simulink model "GridTiedInverterOptimalI_2024_SS"  (R2024a)
settings: Solver=ode23t  StartTime=0  StopTime=0.35  FixedStep=Ts  RelTol=1e-3  EnableMultiTasking=on
PreLoadFcn:
  | GridTiedInverterOptimalIData;
undefined symbols (not defined in the file or in its folder): Ad, Bd, K, Ts, Tsc
libraries: eeTransforms x3, eeLuenbergerObserver x1, eePwmGeneratorTwoLevel x1, eeSinusoidalMeasurement x1, SignalEditorBlockLib x1
CloseFcn:
  | try,close(h1_GridTiedInverterOptimalI),end
  | clear h1_GridTiedInverterOptimalI
  | 
  | 
  | clear simlog_GridTiedInverterOptimalI
  | clear logsout_GridTiedInverterOptimalI
  | 
  | clear Ad Ae Bd Be Cd Ce Dd De Lf Rf
  | clear K L omega Ts  Tsc fsw
Description:
  | Three-Phase Grid-Tied Inverter Optimal Current Control
settings Model: Creator=The MathWorks, Inc.  LastModifiedBy=dilu2
settings SolverCC: AlgebraicLoopSolver=TrustRegion  MaxZcPerStep=1
settings DataIOCC: SaveFormat=Array  SaveOutput=off  SaveTime=off  ReturnWorkspaceOutputs=off  SignalLoggingName=logsout_GridTiedInverterOptimalI
settings OptimizationCC: ReuseModelBlockBuffer=off  ExpressionDepthLimit=2147483647  LifeSpan=inf
settings DebuggingCC: UnconnectedInputMsg=warning  UnconnectedOutputMsg=warning  UnconnectedLineMsg=warning  AllowSymbolicDim=off  StateNameClashWarn=warning  SFUnexpectedBacktrackingDiag=warning  SFNoUnconditionalDefaultTransitionDiag=warning  SFExecutionAtInitializationDiag=none  ArithmeticOperatorsInVariantConditions=warning
settings HardwareCC: ProdBitPerPointer=32  ProdBitPerSizeT=32  ProdBitPerPtrDiffT=32  ProdLargestAtomicFloat=None  ProdIntDivRoundTo=Undefined  ProdEndianess=Unspecified  ProdWordSize=32  ProdHWDeviceType=32-bit Generic
settings ModelReferenceCC: EnableRefExpFcnMdlSchedulingChecks=on  PropagateSignalLabelsOutOfModel=off
settings SFSimCC: SimUseLocalCustomCode=off  CustomCodeUndefinedFunction=UseInterfaceOnly
settings RTWCC: RTWUseLocalCustomCode=off  GPUComputeCapability=3.5  DLArmComputeVersion=19.05
settings CodeAppCC: StateflowObjectComments=on
settings GRTTargetCC: TargetLangStandard=C89/C90 (ANSI)  CombineOutputUpdateFcns=off  GRTInterface=on
settings ConfigComp: CovMetricSettings=dw  CovSaveCumulativeToWorkspaceVar=on  CovSaveSingleToWorkspaceVar=on  CovExternalEMLEnable=off
settings SimscapeCC: SimscapeNormalizeSystem=off  SimscapeLogName=simlog_GridTiedInverterOptimalI

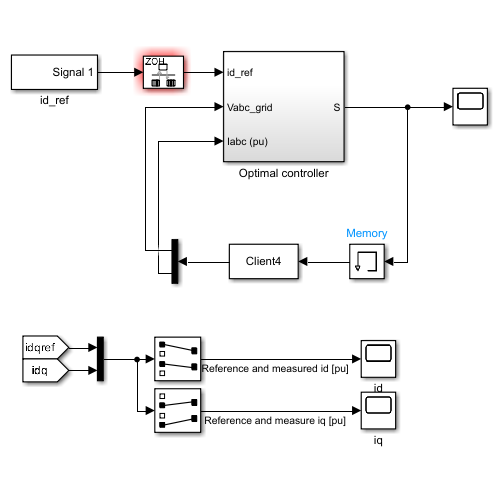
[thumbnail: Simulink's stored preview of the top-level diagram]
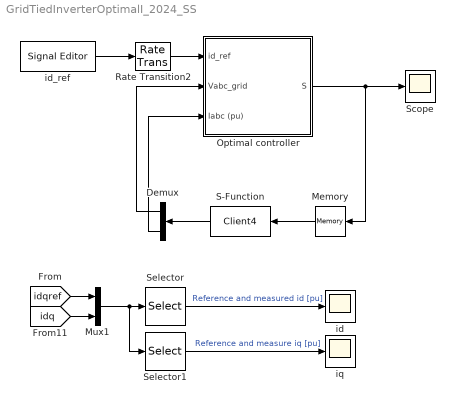
== system GridTiedInverterOptimalI_2024_SS ==
  Demux : Demux  Outputs=2
  Memory : Memory
  Mux1 : Mux  Inputs=2
  Optimal controller : Subsystem
  Rate Transition2 : RateTransition  OutPortSampleTime=Tsc
  S-Function : S-Function  FunctionName=Client4  SFunctionDeploymentMode=off  EnableBusSupport=off
  Scope : Scope
  Selector : Selector  InputPortWidth=4  IndexOptions=Index vector (dialog)  Indices=[1 3]  OutputSizes=1
  Selector1 : Selector  InputPortWidth=4  IndexOptions=Index vector (dialog)  Indices=[2 4]  OutputSizes=1
  id : Scope
  id_ref : SignalEditorBlockLib/Signal Editor  FileName=GridTiedInverterOptimalIIdReference.mat  ActiveScenario=Group_1  ActiveSignal=Signal 1  IsBus=off  OutputBusObjectStr=Bus: BusObject  SampleTime=0  OutputAfterFinalValue=Extrapolation  Unit=inherit  PreserveSignalName=on  ApplySigPropsToAllScenarios=on  ApplySigPropsToAllSignals=off
  iq : Scope
  wires:
  id_ref/1 -> Rate Transition2/1
  Rate Transition2/1 -> Optimal controller/1(id_ref)
  Demux/1 -> Optimal controller/2(Vabc_grid)
  Demux/2 -> Optimal controller/3(Iabc (pu))
  S-Function/1 -> Demux/1
  Optimal controller/1(S) -> Memory/1, Scope/1
  Mux1/1 -> Selector1/1, Selector/1
  Selector/1 -> id/1  "Reference and measured id [pu]"
  [idq] -> Mux1/2
  [idqref] -> Mux1/1
  Selector1/1 -> iq/1  "Reference and measure iq [pu]"
  Memory/1 -> S-Function/1

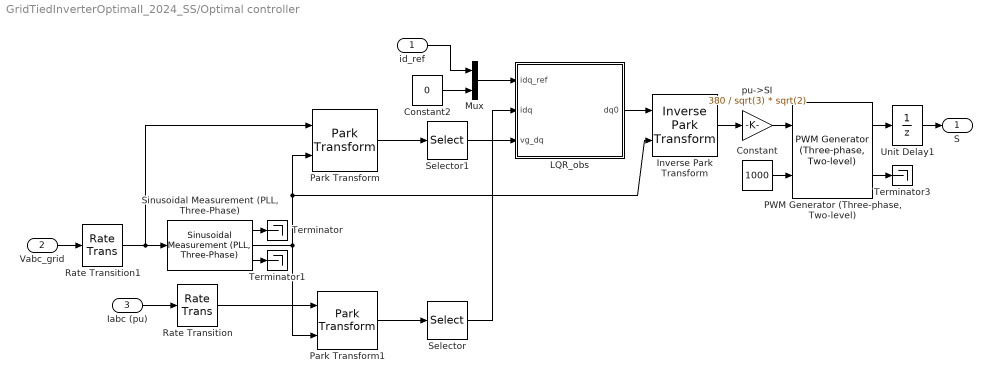
== system GridTiedInverterOptimalI_2024_SS/Optimal controller ==
  id_ref : Inport
  Vabc_grid : Inport  Port=2
  Iabc (pu) : Inport  Port=3
  Constant : Constant  Value=1000
  Constant2 : Constant  Value=0  SampleTime=Tsc
  Inverse Park Transform : eeTransforms/Inverse Park Transform  AxisAlignment=Q-axis  PowerInvariant=off
  LQR_obs : Subsystem
  Mux : Mux  Inputs=2
  "PWM Generator (Three-phase, Two-level)" : eePwmGeneratorTwoLevel/PWM Generator (Three-phase, Two-level)  PWMMode=Continuous PWM (CPWM)  CPWMMode=SPWM: sinusoidal PWM  DPWMMode=60 DPWM: 60 degree discontinuous PWM  fsw=10000  Ts=Ts
  Park Transform : eeTransforms/Park Transform  AxisAlignment=Q-axis  PowerInvariant=off
  Park Transform1 : eeTransforms/Park Transform  AxisAlignment=Q-axis  PowerInvariant=off
  Rate Transition : RateTransition  OutPortSampleTime=Tsc
  Rate Transition1 : RateTransition  OutPortSampleTime=Tsc
  Selector : Selector  InputPortWidth=3  IndexOptions=Index vector (dialog)  Indices=[1 2]  OutputSizes=1
  Selector1 : Selector  InputPortWidth=3  IndexOptions=Index vector (dialog)  Indices=[1 2]  OutputSizes=1
  "Sinusoidal Measurement (PLL, Three-Phase)" : eeSinusoidalMeasurement/Sinusoidal Measurement (PLL, Three-Phase)  Kp_LF=150  Ki_LF=150  F0=60  Theta0=0  Ts=Tsc
  Terminator : Terminator
  Terminator1 : Terminator
  Terminator3 : Terminator
  Unit Delay1 : UnitDelay  SampleTime=Ts  HasFrameUpgradeWarning=on
  pu->SI : Gain  Gain=380 / sqrt(3) * sqrt(2)
  S : Outport
  wires:
  Vabc_grid/1 -> Rate Transition1/1
  Mux/1 -> LQR_obs/1(idq_ref)
  Selector/1 -> LQR_obs/2(idq)
  LQR_obs/1(dq0) -> Inverse Park Transform/1
  Iabc (pu)/1 -> Rate Transition/1
  Park Transform1/1 -> Selector/1
  Selector1/1 -> LQR_obs/3(vg_dq)
  "Sinusoidal Measurement (PLL, Three-Phase)"/2 -> Park Transform/2, Inverse Park Transform/2, Park Transform1/2
  "Sinusoidal Measurement (PLL, Three-Phase)"/1 -> Terminator/1
  "Sinusoidal Measurement (PLL, Three-Phase)"/3 -> Terminator1/1
  "PWM Generator (Three-phase, Two-level)"/2 -> Terminator3/1
  Constant/1 -> "PWM Generator (Three-phase, Two-level)"/2
  Inverse Park Transform/1 -> pu->SI/1
  "PWM Generator (Three-phase, Two-level)"/1 -> Unit Delay1/1
  Unit Delay1/1 -> S/1
  Park Transform/1 -> Selector1/1
  Constant2/1 -> Mux/2
  Rate Transition/1 -> Park Transform1/1
  Rate Transition1/1 -> Park Transform/1, "Sinusoidal Measurement (PLL, Three-Phase)"/1
  id_ref/1 -> Mux/1
  pu->SI/1 -> "PWM Generator (Three-phase, Two-level)"/1

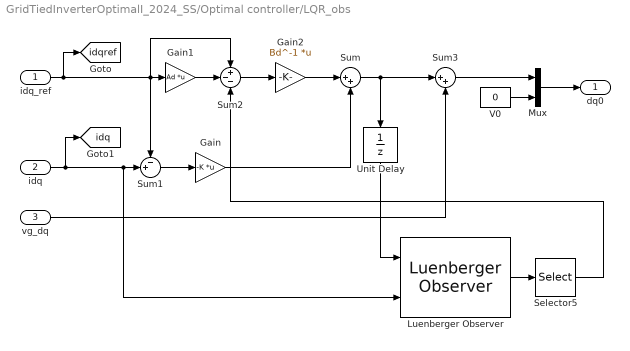
== system GridTiedInverterOptimalI_2024_SS/Optimal controller/LQR_obs ==
  idq_ref : Inport
  idq : Inport  Port=2
  vg_dq : Inport  Port=3
  Gain : Gain  Gain=-K  Multiplication=Matrix(K*u)
  Gain1 : Gain  Gain=Ad  Multiplication=Matrix(K*u)
  Gain2 : Gain  Gain=Bd^-1  Multiplication=Matrix(K*u)
  Luenberger Observer : eeLuenbergerObserver/Luenberger Observer  StateSpaceType=Discrete-time  Ad=Ae  Bd=Be  Cd=Ce  Dd=De  A=1  B=1  C=1  D=1  ObserverDesign=Observer gain  Ld=L  DesiredEigenvalues=0  x0=[0;0;0;0]  Tsd=0.1  Ts=Tsc
  Mux : Mux  Inputs=2
  Selector5 : Selector  InputPortWidth=4  IndexOptions=Index vector (dialog)  Indices=[3 4]  OutputSizes=1
  Sum : Sum  Inputs=|++
  Sum1 : Sum  Inputs=-+|
  Sum2 : Sum  Inputs=+--
  Sum3 : Sum  Inputs=|++
  Unit Delay : UnitDelay  SampleTime=-1  HasFrameUpgradeWarning=on
  V0 : Constant  Value=0
  dq0 : Outport
  tag scope: idq=global, idqref=global
  wires:
  idq_ref/1 -> Sum2/1, Sum1/1, Gain1/1, [idqref]
  Gain1/1 -> Sum2/2
  Luenberger Observer/1 -> Selector5/1
  Sum2/1 -> Gain2/1
  Gain2/1 -> Sum/1
  idq/1 -> [idq], Luenberger Observer/2, Sum1/2
  Sum1/1 -> Gain/1
  Gain/1 -> Sum/2
  Sum/1 -> Unit Delay/1, Sum3/1
  Sum3/1 -> Mux/1
  V0/1 -> Mux/2
  Mux/1 -> dq0/1
  vg_dq/1 -> Sum3/2
  Selector5/1 -> Sum2/3
  Unit Delay/1 -> Luenberger Observer/1
